simulink model "sysgenSynthFSE"  (Simulink 7.2)
settings: Solver=ode45  StartTime=0.0  StopTime=1780  RelTol=1e-3
values from neighbouring files (symbols this model uses):
  j = find(xLabel==')')    [sdspfscope2_r13.m]
undefined symbols (not defined in the file or in its folder): xlsfunxy
libraries: xbsIndex_r4 x72, dspsigops x2, dspmlti4 x2, xbsCopyrightNotice_r4 x1, dspsnks4 x1, dspbuff3 x1
(part 2 of 2)

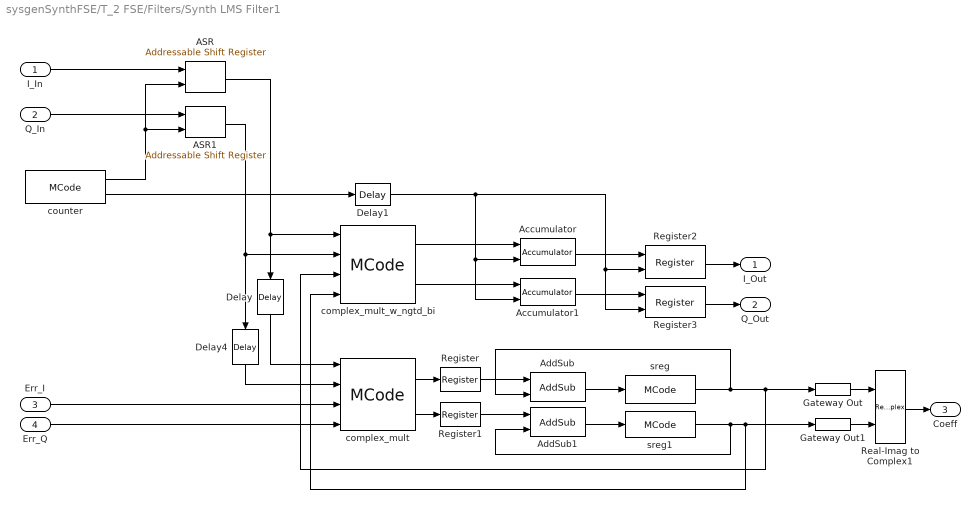
== system sysgenSynthFSE/T_2 FSE/Filters/Synth LMS Filter1 ==
  I_In : Inport  OutDataType=sfix(16)  OutScaling=2^0
  Q_In : Inport  Port=2  OutDataType=sfix(16)  OutScaling=2^0
  Err_I : Inport  Port=3  OutDataType=sfix(16)  OutScaling=2^0
  Err_Q : Inport  Port=4  OutDataType=sfix(16)  OutScaling=2^0
  ASR : xbsIndex_r4/Addressable Shift Register  infer_latency=off  depth=4  initVector=[0]  en=off  dbl_ovrd=off  use_behavioral_HDL=on  use_rpm=on  block_type=addrsr
      settings: infoedit="Delay of configurable length.  Any element in the delay line can be addressed and driven onto the output port.<P><P>Hardware notes: Implemented using SRL16s.  If a Virtex-II device is used, multiple SRLC16s are cascaded together."  block_version=VER_STRING_GOES_HERE
  ASR1 : xbsIndex_r4/Addressable Shift Register  infer_latency=off  depth=4  initVector=[0]  en=off  dbl_ovrd=off  use_behavioral_HDL=on  use_rpm=on  block_type=addrsr
      settings: infoedit="Delay of configurable length.  Any element in the delay line can be addressed and driven onto the output port.<P><P>Hardware notes: Implemented using SRL16s.  If a Virtex-II device is used, multiple SRLC16s are cascaded together."  block_version=VER_STRING_GOES_HERE
  Accumulator : xbsIndex_r4/Accumulator  operation=Add  n_bits=36  overflow=Wrap  scale=1  rst=on  hasbypass=off  en=off  dbl_ovrd=off  use_behavioral_HDL=on  implementation=Fabric  block_type=accum
      settings: infoedit="Adder or subtractor-based accumulator.   Output type and binary point position match the input.<P><P>Hardware notes: When \"Reinitialize with Input 'b' on Reset\" is selected, the accumulator is forced to run at the system rate even if the input 'b' is running at a slower rate."  block_version=VER_STRING_GOES_HERE
  Accumulator1 : xbsIndex_r4/Accumulator  operation=Add  n_bits=36  overflow=Wrap  scale=1  rst=on  hasbypass=off  en=off  dbl_ovrd=off  use_behavioral_HDL=on  implementation=Fabric  block_type=accum
      settings: infoedit="Adder or subtractor-based accumulator.   Output type and binary point position match the input.<P><P>Hardware notes: When \"Reinitialize with Input 'b' on Reset\" is selected, the accumulator is forced to run at the system rate even if the input 'b' is running at a slower rate."  block_version=VER_STRING_GOES_HERE
  AddSub : xbsIndex_r4/AddSub  mode=Addition  use_carryin=off  use_carryout=off  en=off  latency=0  precision=User Defined  arith_type="Signed  (2's comp)"  n_bits=18  bin_pt=10  quantization="Round  (unbiased: +/- Inf)"  overflow=Saturate  dbl_ovrd=off  use_behavioral_HDL=on  hw_selection=Fabric  pipelined=off  use_rpm=on  block_type=addsub
      settings: block_version=VER_STRING_GOES_HERE
  AddSub1 : xbsIndex_r4/AddSub  mode=Addition  use_carryin=off  use_carryout=off  en=off  latency=0  precision=User Defined  arith_type="Signed  (2's comp)"  n_bits=18  bin_pt=10  quantization="Round  (unbiased: +/- Inf)"  overflow=Saturate  dbl_ovrd=off  use_behavioral_HDL=on  hw_selection=Fabric  pipelined=off  use_rpm=on  block_type=addsub
      settings: block_version=VER_STRING_GOES_HERE
  Delay : xbsIndex_r4/Delay  Orientation=down  en=off  latency=27  dbl_ovrd=off  reg_retiming=off  block_type=delay
      settings: infoedit="Delay line having  configurable length.<P><P>Hardware notes: A delay line is a chain, each link of which is an SRL16 followed by a flip-flop. If register retiming is enabled, the delay line is a chain of flip-flops."  xl_area=[12 24 0 24 0 0 0]  block_version=VER_STRING_GOES_HERE
  Delay1 : xbsIndex_r4/Delay  en=off  latency=3  dbl_ovrd=off  reg_retiming=on  block_type=delay
      settings: infoedit="Delay line having  configurable length.<P><P>Hardware notes: A delay line is a chain, each link of which is an SRL16 followed by a flip-flop. If register retiming is enabled, the delay line is a chain of flip-flops."  xl_area=[1 1 0 1 0 0 0]  block_version=VER_STRING_GOES_HERE
  Delay4 : xbsIndex_r4/Delay  Orientation=down  en=off  latency=27  dbl_ovrd=off  reg_retiming=off  block_type=delay
      settings: infoedit="Delay line having  configurable length.<P><P>Hardware notes: A delay line is a chain, each link of which is an SRL16 followed by a flip-flop. If register retiming is enabled, the delay line is a chain of flip-flops."  xl_area=[12 24 0 24 0 0 0]  block_version=VER_STRING_GOES_HERE
  Gateway Out : xbsIndex_r4/Gateway Out  hdl_port=off  timing_constraint=None  locs_specified=off  LOCs={}  block_type=gatewayout
      settings: infoedit="Gateway out block.  Converts Xilinx fixed point inputs into ouputs of type Simulink integer, double, or fixed point.<P><P>Hardware notes:  In hardware these blocks become top level output ports or are discarded, depending on how they are configured."  xl_area=[0 0 0 0 0 0 0]  block_version=VER_STRING_GOES_HERE
  Gateway Out1 : xbsIndex_r4/Gateway Out  hdl_port=off  timing_constraint=None  locs_specified=off  LOCs={}  block_type=gatewayout
      settings: infoedit="Gateway out block.  Converts Xilinx fixed point inputs into ouputs of type Simulink integer, double, or fixed point.<P><P>Hardware notes:  In hardware these blocks become top level output ports or are discarded, depending on how they are configured."  xl_area=[0 0 0 0 0 0 0]  block_version=VER_STRING_GOES_HERE
  Real-Imag to Complex1 : RealImagToComplex
  Register : xbsIndex_r4/Register  init=0  rst=off  en=off  dbl_ovrd=off  block_type=register
      settings: xl_area=[18 36 0 0 0 0 0]  block_version=VER_STRING_GOES_HERE
  Register1 : xbsIndex_r4/Register  init=0  rst=off  en=off  dbl_ovrd=off  block_type=register
      settings: xl_area=[18 36 0 0 0 0 0]  block_version=VER_STRING_GOES_HERE
  Register2 : xbsIndex_r4/Register  init=0  rst=off  en=on  dbl_ovrd=off  block_type=register
      settings: xl_area=[18 36 0 0 0 0 0]  block_version=VER_STRING_GOES_HERE
  Register3 : xbsIndex_r4/Register  init=0  rst=off  en=on  dbl_ovrd=off  block_type=register
      settings: xl_area=[18 36 0 0 0 0 0]  block_version=VER_STRING_GOES_HERE
  complex_mult : xbsIndex_r4/MCode  mfname=complex_mult  explicit_period=off  period=1  dbl_ovrd=off  enable_stdout=off  enable_debug=off  suppress_output=off  defparams={'negate_bi', 0}  hide_port_list={}  block_type=mcode
      settings: xl_area=[0, 0, 0, 0, 0, 0, 0]  block_version=8.1
  complex_mult_w_ngtd_bi : xbsIndex_r4/MCode  mfname=complex_mult  explicit_period=off  period=1  dbl_ovrd=off  enable_stdout=off  enable_debug=off  suppress_output=off  defparams={'negate_bi', 1}  hide_port_list={}  block_type=mcode
      settings: xl_area=[0, 0, 0, 0, 0, 0, 0]  block_version=8.1
  counter : xbsIndex_r4/MCode  mfname=fir_fsm  explicit_period=on  period=1  dbl_ovrd=off  enable_stdout=off  enable_debug=off  suppress_output=off  defparams={'reset', false,'init', 3}  hide_port_list={}  block_type=mcode
      settings: xl_area=[0, 0, 0, 0, 0, 0, 0]  block_version=8.1
  sreg : xbsIndex_r4/MCode  mfname=sreg  explicit_period=off  period=1  dbl_ovrd=off  enable_stdout=off  enable_debug=off  suppress_output=off  defparams={'len',4,'init',init_i}  hide_port_list={}  block_type=mcode
      settings: xl_area=[0, 0, 0, 0, 0, 0, 0]  block_version=8.1
  sreg1 : xbsIndex_r4/MCode  mfname=sreg  explicit_period=off  period=1  dbl_ovrd=off  enable_stdout=off  enable_debug=off  suppress_output=off  defparams={'len',4,'init',init_q}  hide_port_list={}  block_type=mcode
      settings: xl_area=[0, 0, 0, 0, 0, 0, 0]  block_version=8.1
  I_Out : Outport  OutDataType=sfix(16)  OutScaling=2^0
  Q_Out : Outport  Port=2  OutDataType=sfix(16)  OutScaling=2^0
  Coeff : Outport  Port=3  OutDataType=sfix(16)  OutScaling=2^0
  wires:
  sreg1/1 -> AddSub1/2, Gateway Out1/1, complex_mult_w_ngtd_bi/4
  Delay4/1 -> complex_mult/2
  Delay/1 -> complex_mult/1
  Accumulator/1 -> Register2/1
  Delay1/1 -> Accumulator1/2, Accumulator/2, Register2/2, Register3/2
  complex_mult_w_ngtd_bi/1 -> Accumulator/1
  complex_mult_w_ngtd_bi/2 -> Accumulator1/1
  Accumulator1/1 -> Register3/1
  Register1/1 -> AddSub1/1
  Register/1 -> AddSub/1
  sreg/1 -> AddSub/2, Gateway Out/1, complex_mult_w_ngtd_bi/3
  counter/2 -> Delay1/1
  counter/1 -> ASR1/2, ASR/2
  AddSub1/1 -> sreg1/1
  AddSub/1 -> sreg/1
  Gateway Out/1 -> Real-Imag to Complex1/1
  Gateway Out1/1 -> Real-Imag to Complex1/2
  Real-Imag to Complex1/1 -> Coeff/1
  Err_I/1 -> complex_mult/3
  Err_Q/1 -> complex_mult/4
  complex_mult/2 -> Register1/1
  complex_mult/1 -> Register/1
  Register2/1 -> I_Out/1
  Register3/1 -> Q_Out/1
  ASR/1 -> Delay/1, complex_mult_w_ngtd_bi/1
  ASR1/1 -> Delay4/1, complex_mult_w_ngtd_bi/2
  I_In/1 -> ASR/1
  Q_In/1 -> ASR1/1
